simulink model "rocky_closed_loop"  (R2022b)
settings: Solver=VariableStepAuto  StartTime=0.0  StopTime=20  RelTol=1e-3
model workspace (MAT data in the model file):
  Ci = -719.58
  Cp = 0
  Ji = -1025.4
  Jp = 78.59
  K = 0.00333
  Ki = 11064
  Kp = 2670.4
  g = 9.81
  l = 0.5836
  tau = 0.0505
settings Model: Creator=ali1  LastModifiedBy=ali1

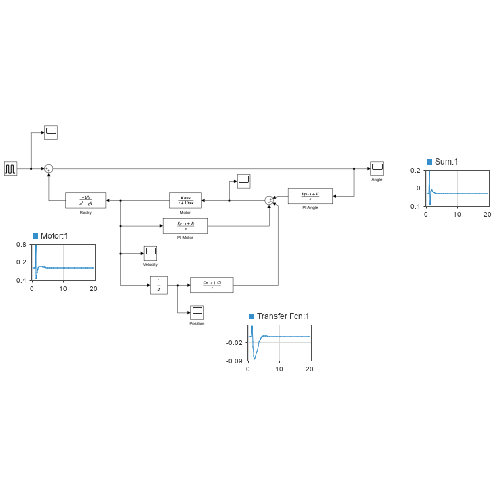
[thumbnail: Simulink's stored preview of the top-level diagram]
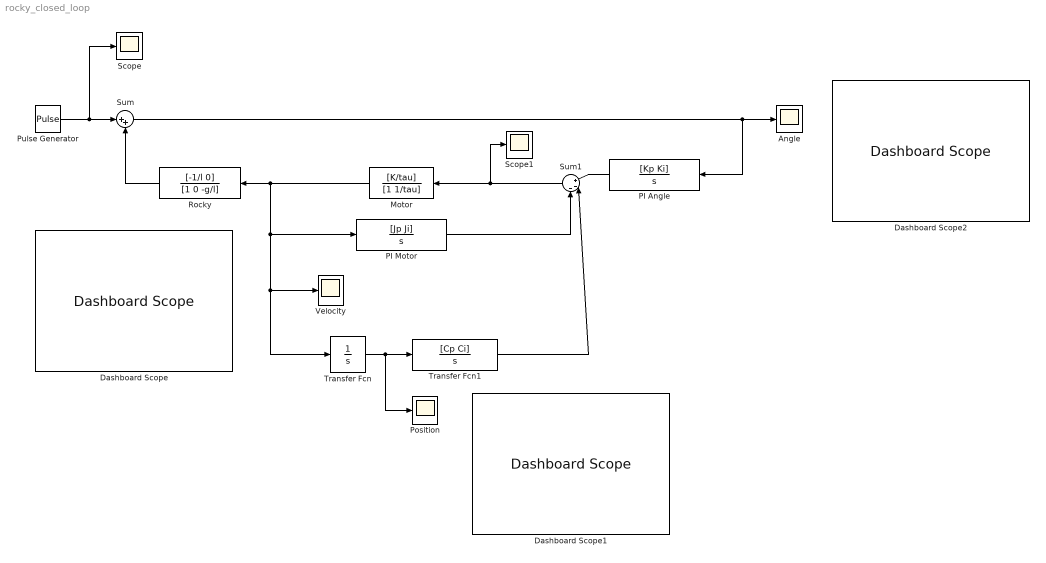
== system rocky_closed_loop ==
  Angle : Scope
  Dashboard Scope : DashboardScope
  Dashboard Scope1 : DashboardScope
  Dashboard Scope2 : DashboardScope
  Motor : TransferFcn  Numerator=[K/tau]  Denominator=[1 1/tau]
  PI Angle : TransferFcn  Numerator=[Kp Ki]  Denominator=[1 0]
  PI Motor : TransferFcn  Numerator=[Jp Ji]  Denominator=[1 0]
  Position : Scope
  Pulse Generator : DiscretePulseGenerator  PulseType=Time based  Amplitude=.15  Period=20  PulseWidth=.25  PhaseDelay=1
  Rocky : TransferFcn  Numerator=[-1/l 0]  Denominator=[1 0 -g/l]
  Scope : Scope
  Scope1 : Scope
  Sum : Sum  Inputs=|++
  Sum1 : Sum  Inputs=|+--
  Transfer Fcn : TransferFcn  Denominator=[1 0]
  Transfer Fcn1 : TransferFcn  Numerator=[Cp Ci]  Denominator=[1 0]
  Velocity : Scope
  wires:
  Pulse Generator/1 -> Scope/1, Sum/1
  Rocky/1 -> Sum/2
  Motor/1 -> Transfer Fcn/1, Velocity/1, PI Motor/1, Rocky/1
  Sum/1 -> PI Angle/1, Angle/1
  Sum1/1 -> Scope1/1, Motor/1
  PI Angle/1 -> Sum1/1
  Transfer Fcn/1 -> Position/1, Transfer Fcn1/1
  Transfer Fcn1/1 -> Sum1/2
  PI Motor/1 -> Sum1/3
